simulink model "sm_car_testrig_susp_splitla_shockf_hp"  (R2026a)
settings: Solver=ode23t  StopTime=1e-9  MaxStep=1e-3  AbsTol=1e-4  EnableMultiTasking=on
PostLoadFcn:
  | sm_car_load_vehicle_data(bdroot,'032');
undefined symbols (not defined in the file): Init, UAf, UAr, Vehicle, X, Y, Z
libraries: sm_lib x125, nesl_utility x73, Linkage_Arms x8, Suspension_Utilities x6, fl_lib x4, Linkage_SpLA_S2LAF x2, Linkage_Shock x2, Linkage_Uprights x2
(part 2 of 5)

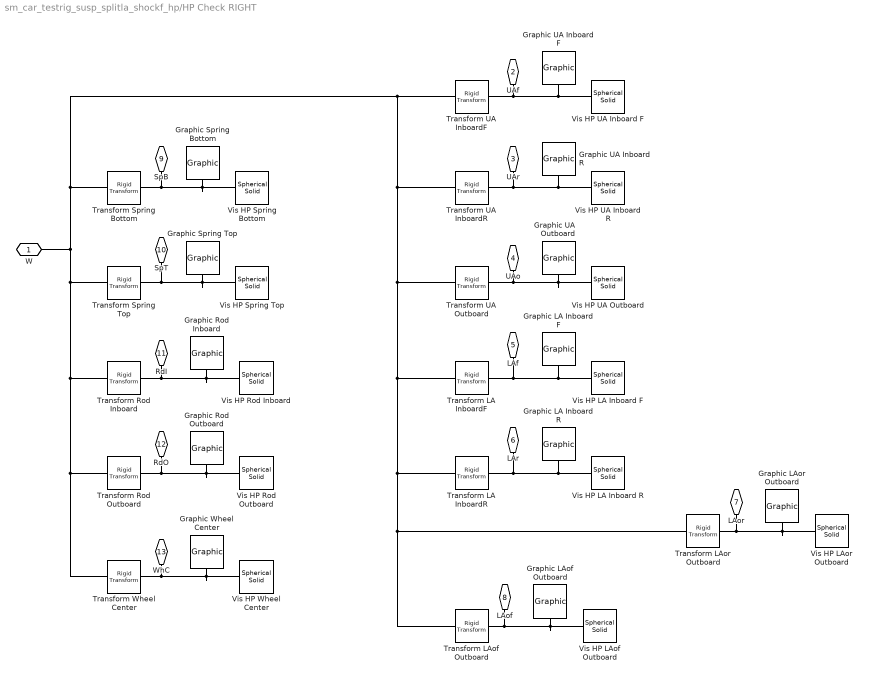
== system sm_car_testrig_susp_splitla_shockf_hp/HP Check RIGHT ==
  Graphic LA Inboard F : sm_lib/Body Elements/Graphic  GraphicType=Marker  MarkerShape=Frame  MarkerSize=size_frm_vis  GraphicVisPropType=SimpleVisualProperties  GraphicDiffuseColor=clr_frm_vis  GraphicOpacity=opc_frm_vis  GraphicSpecularColor=[0.5 0.5 0.5 1.0]  GraphicAmbientColor=[0.15 0.15 0.15 1.0]  GraphicEmissiveColor=[0.0 0.0 0.0 1.0]  GraphicShininess=75
  Graphic LA Inboard R : sm_lib/Body Elements/Graphic  GraphicType=Marker  MarkerShape=Frame  MarkerSize=size_frm_vis  GraphicVisPropType=SimpleVisualProperties  GraphicDiffuseColor=clr_frm_vis  GraphicOpacity=opc_frm_vis  GraphicSpecularColor=[0.5 0.5 0.5 1.0]  GraphicAmbientColor=[0.15 0.15 0.15 1.0]  GraphicEmissiveColor=[0.0 0.0 0.0 1.0]  GraphicShininess=75
  Graphic LAof Outboard : sm_lib/Body Elements/Graphic  GraphicType=Marker  MarkerShape=Frame  MarkerSize=size_frm_vis  GraphicVisPropType=SimpleVisualProperties  GraphicDiffuseColor=clr_frm_vis  GraphicOpacity=opc_frm_vis  GraphicSpecularColor=[0.5 0.5 0.5 1.0]  GraphicAmbientColor=[0.15 0.15 0.15 1.0]  GraphicEmissiveColor=[0.0 0.0 0.0 1.0]  GraphicShininess=75
  Graphic LAor Outboard : sm_lib/Body Elements/Graphic  GraphicType=Marker  MarkerShape=Frame  MarkerSize=size_frm_vis  GraphicVisPropType=SimpleVisualProperties  GraphicDiffuseColor=clr_frm_vis  GraphicOpacity=opc_frm_vis  GraphicSpecularColor=[0.5 0.5 0.5 1.0]  GraphicAmbientColor=[0.15 0.15 0.15 1.0]  GraphicEmissiveColor=[0.0 0.0 0.0 1.0]  GraphicShininess=75
  Graphic Rod Inboard : sm_lib/Body Elements/Graphic  GraphicType=Marker  MarkerShape=Frame  MarkerSize=size_frm_vis  GraphicVisPropType=SimpleVisualProperties  GraphicDiffuseColor=clr_frm_vis  GraphicOpacity=opc_frm_vis  GraphicSpecularColor=[0.5 0.5 0.5 1.0]  GraphicAmbientColor=[0.15 0.15 0.15 1.0]  GraphicEmissiveColor=[0.0 0.0 0.0 1.0]  GraphicShininess=75
  Graphic Rod Outboard : sm_lib/Body Elements/Graphic  GraphicType=Marker  MarkerShape=Frame  MarkerSize=size_frm_vis  GraphicVisPropType=SimpleVisualProperties  GraphicDiffuseColor=clr_frm_vis  GraphicOpacity=opc_frm_vis  GraphicSpecularColor=[0.5 0.5 0.5 1.0]  GraphicAmbientColor=[0.15 0.15 0.15 1.0]  GraphicEmissiveColor=[0.0 0.0 0.0 1.0]  GraphicShininess=75
  Graphic Spring Bottom : sm_lib/Body Elements/Graphic  GraphicType=Marker  MarkerShape=Frame  MarkerSize=size_frm_vis  GraphicVisPropType=SimpleVisualProperties  GraphicDiffuseColor=clr_frm_vis  GraphicOpacity=opc_frm_vis  GraphicSpecularColor=[0.5 0.5 0.5 1.0]  GraphicAmbientColor=[0.15 0.15 0.15 1.0]  GraphicEmissiveColor=[0.0 0.0 0.0 1.0]  GraphicShininess=75
  Graphic Spring Top : sm_lib/Body Elements/Graphic  GraphicType=Marker  MarkerShape=Frame  MarkerSize=size_frm_vis  GraphicVisPropType=SimpleVisualProperties  GraphicDiffuseColor=clr_frm_vis  GraphicOpacity=opc_frm_vis  GraphicSpecularColor=[0.5 0.5 0.5 1.0]  GraphicAmbientColor=[0.15 0.15 0.15 1.0]  GraphicEmissiveColor=[0.0 0.0 0.0 1.0]  GraphicShininess=75
  Graphic UA Inboard F : sm_lib/Body Elements/Graphic  GraphicType=Marker  MarkerShape=Frame  MarkerSize=size_frm_vis  GraphicVisPropType=SimpleVisualProperties  GraphicDiffuseColor=clr_frm_vis  GraphicOpacity=opc_frm_vis  GraphicSpecularColor=[0.5 0.5 0.5 1.0]  GraphicAmbientColor=[0.15 0.15 0.15 1.0]  GraphicEmissiveColor=[0.0 0.0 0.0 1.0]  GraphicShininess=75
  Graphic UA Inboard R : sm_lib/Body Elements/Graphic  GraphicType=Marker  MarkerShape=Frame  MarkerSize=size_frm_vis  GraphicVisPropType=SimpleVisualProperties  GraphicDiffuseColor=clr_frm_vis  GraphicOpacity=opc_frm_vis  GraphicSpecularColor=[0.5 0.5 0.5 1.0]  GraphicAmbientColor=[0.15 0.15 0.15 1.0]  GraphicEmissiveColor=[0.0 0.0 0.0 1.0]  GraphicShininess=75
  Graphic UA Outboard : sm_lib/Body Elements/Graphic  GraphicType=Marker  MarkerShape=Frame  MarkerSize=size_frm_vis  GraphicVisPropType=SimpleVisualProperties  GraphicDiffuseColor=clr_frm_vis  GraphicOpacity=opc_frm_vis  GraphicSpecularColor=[0.5 0.5 0.5 1.0]  GraphicAmbientColor=[0.15 0.15 0.15 1.0]  GraphicEmissiveColor=[0.0 0.0 0.0 1.0]  GraphicShininess=75
  Graphic Wheel Center : sm_lib/Body Elements/Graphic  GraphicType=Marker  MarkerShape=Frame  MarkerSize=size_frm_vis  GraphicVisPropType=SimpleVisualProperties  GraphicDiffuseColor=clr_frm_vis  GraphicOpacity=opc_frm_vis  GraphicSpecularColor=[0.5 0.5 0.5 1.0]  GraphicAmbientColor=[0.15 0.15 0.15 1.0]  GraphicEmissiveColor=[0.0 0.0 0.0 1.0]  GraphicShininess=75
  Transform LA InboardF : sm_lib/Frames and Transforms/Rigid Transform  RotationMethod=None  FollAlignAxisA=+X  BaseAlignAxisA=+Y  FollAlignAxisB=+Y  BaseAlignAxisB=+Z  RotationStandardAxis=+Z  RotationAngle=0.0  RotationAngleUnits=deg  RotationArbitraryAxis=[0 0 1]  RotationSequenceAxes=FollowerAxes  RotationSequence=XYX  RotationSequenceAngles=[0 0 0]  RotationSequenceAnglesUnits=deg  RotationMatrix=[1 0 0; 0 1 0; 0 0 1]  Quaternion=[1 0 0 0]  TranslationMethod=Cartesian  TranslationCartesianOffset=Linkage.LowerArmF.sInboard.Value.*rhs_hp  TranslationCartesianOffsetUnits=m  TranslationStandardAxis=+Z  TranslationStandardOffset=0  TranslationStandardOffsetUnits=m  TranslationROffset=0  TranslationROffsetUnits=m  TranslationThetaOffset=0  TranslationThetaOffsetUnits=deg  TranslationZOffset=0  TranslationZOffsetUnits=m
      settings: AttributesFormatString=%<TranslationCartesianOffset>
  Transform LA InboardR : sm_lib/Frames and Transforms/Rigid Transform  RotationMethod=None  FollAlignAxisA=+X  BaseAlignAxisA=+Y  FollAlignAxisB=+Y  BaseAlignAxisB=+Z  RotationStandardAxis=+Z  RotationAngle=0.0  RotationAngleUnits=deg  RotationArbitraryAxis=[0 0 1]  RotationSequenceAxes=FollowerAxes  RotationSequence=XYX  RotationSequenceAngles=[0 0 0]  RotationSequenceAnglesUnits=deg  RotationMatrix=[1 0 0; 0 1 0; 0 0 1]  Quaternion=[1 0 0 0]  TranslationMethod=Cartesian  TranslationCartesianOffset=Linkage.LowerArmR.sInboard.Value.*rhs_hp  TranslationCartesianOffsetUnits=m  TranslationStandardAxis=+Z  TranslationStandardOffset=0  TranslationStandardOffsetUnits=m  TranslationROffset=0  TranslationROffsetUnits=m  TranslationThetaOffset=0  TranslationThetaOffsetUnits=deg  TranslationZOffset=0  TranslationZOffsetUnits=m
      settings: AttributesFormatString=%<TranslationCartesianOffset>
  Transform LAof Outboard : sm_lib/Frames and Transforms/Rigid Transform  RotationMethod=None  FollAlignAxisA=+X  BaseAlignAxisA=+Y  FollAlignAxisB=+Y  BaseAlignAxisB=+Z  RotationStandardAxis=+Z  RotationAngle=0.0  RotationAngleUnits=deg  RotationArbitraryAxis=[0 0 1]  RotationSequenceAxes=FollowerAxes  RotationSequence=XYX  RotationSequenceAngles=[0 0 0]  RotationSequenceAnglesUnits=deg  RotationMatrix=[1 0 0; 0 1 0; 0 0 1]  Quaternion=[1 0 0 0]  TranslationMethod=Cartesian  TranslationCartesianOffset=Linkage.LowerArmF.sOutboard.Value.*rhs_hp  TranslationCartesianOffsetUnits=m  TranslationStandardAxis=+Z  TranslationStandardOffset=0  TranslationStandardOffsetUnits=m  TranslationROffset=0  TranslationROffsetUnits=m  TranslationThetaOffset=0  TranslationThetaOffsetUnits=deg  TranslationZOffset=0  TranslationZOffsetUnits=m
      settings: AttributesFormatString=%<TranslationCartesianOffset>
  Transform LAor Outboard : sm_lib/Frames and Transforms/Rigid Transform  RotationMethod=None  FollAlignAxisA=+X  BaseAlignAxisA=+Y  FollAlignAxisB=+Y  BaseAlignAxisB=+Z  RotationStandardAxis=+Z  RotationAngle=0.0  RotationAngleUnits=deg  RotationArbitraryAxis=[0 0 1]  RotationSequenceAxes=FollowerAxes  RotationSequence=XYX  RotationSequenceAngles=[0 0 0]  RotationSequenceAnglesUnits=deg  RotationMatrix=[1 0 0; 0 1 0; 0 0 1]  Quaternion=[1 0 0 0]  TranslationMethod=Cartesian  TranslationCartesianOffset=Linkage.LowerArmR.sOutboard.Value.*rhs_hp  TranslationCartesianOffsetUnits=m  TranslationStandardAxis=+Z  TranslationStandardOffset=0  TranslationStandardOffsetUnits=m  TranslationROffset=0  TranslationROffsetUnits=m  TranslationThetaOffset=0  TranslationThetaOffsetUnits=deg  TranslationZOffset=0  TranslationZOffsetUnits=m
      settings: AttributesFormatString=%<TranslationCartesianOffset>
  Transform Rod Inboard : sm_lib/Frames and Transforms/Rigid Transform  RotationMethod=None  FollAlignAxisA=+X  BaseAlignAxisA=+Y  FollAlignAxisB=+Y  BaseAlignAxisB=+Z  RotationStandardAxis=+Z  RotationAngle=0.0  RotationAngleUnits=deg  RotationArbitraryAxis=[0 0 1]  RotationSequenceAxes=FollowerAxes  RotationSequence=XYX  RotationSequenceAngles=[0 0 0]  RotationSequenceAnglesUnits=deg  RotationMatrix=[1 0 0; 0 1 0; 0 0 1]  Quaternion=[1 0 0 0]  TranslationMethod=Cartesian  TranslationCartesianOffset=Linkage.TrackRod.sInboard.Value.*rhs_hp  TranslationCartesianOffsetUnits=m  TranslationStandardAxis=+Z  TranslationStandardOffset=0  TranslationStandardOffsetUnits=m  TranslationROffset=0  TranslationROffsetUnits=m  TranslationThetaOffset=0  TranslationThetaOffsetUnits=deg  TranslationZOffset=0  TranslationZOffsetUnits=m
      settings: AttributesFormatString=%<TranslationCartesianOffset>
  Transform Rod Outboard : sm_lib/Frames and Transforms/Rigid Transform  RotationMethod=None  FollAlignAxisA=+X  BaseAlignAxisA=+Y  FollAlignAxisB=+Y  BaseAlignAxisB=+Z  RotationStandardAxis=+Z  RotationAngle=0.0  RotationAngleUnits=deg  RotationArbitraryAxis=[0 0 1]  RotationSequenceAxes=FollowerAxes  RotationSequence=XYX  RotationSequenceAngles=[0 0 0]  RotationSequenceAnglesUnits=deg  RotationMatrix=[1 0 0; 0 1 0; 0 0 1]  Quaternion=[1 0 0 0]  TranslationMethod=Cartesian  TranslationCartesianOffset=Linkage.TrackRod.sOutboard.Value.*rhs_hp  TranslationCartesianOffsetUnits=m  TranslationStandardAxis=+Z  TranslationStandardOffset=0  TranslationStandardOffsetUnits=m  TranslationROffset=0  TranslationROffsetUnits=m  TranslationThetaOffset=0  TranslationThetaOffsetUnits=deg  TranslationZOffset=0  TranslationZOffsetUnits=m
      settings: AttributesFormatString=%<TranslationCartesianOffset>
  Transform Spring Bottom : sm_lib/Frames and Transforms/Rigid Transform  RotationMethod=None  FollAlignAxisA=+X  BaseAlignAxisA=+Y  FollAlignAxisB=+Y  BaseAlignAxisB=+Z  RotationStandardAxis=+Z  RotationAngle=0.0  RotationAngleUnits=deg  RotationArbitraryAxis=[0 0 1]  RotationSequenceAxes=FollowerAxes  RotationSequence=XYX  RotationSequenceAngles=[0 0 0]  RotationSequenceAnglesUnits=deg  RotationMatrix=[1 0 0; 0 1 0; 0 0 1]  Quaternion=[1 0 0 0]  TranslationMethod=Cartesian  TranslationCartesianOffset=Linkage.Shock.sBottom.Value.*rhs_hp  TranslationCartesianOffsetUnits=m  TranslationStandardAxis=+Z  TranslationStandardOffset=0  TranslationStandardOffsetUnits=m  TranslationROffset=0  TranslationROffsetUnits=m  TranslationThetaOffset=0  TranslationThetaOffsetUnits=deg  TranslationZOffset=0  TranslationZOffsetUnits=m
      settings: AttributesFormatString=%<TranslationCartesianOffset>
  Transform Spring Top : sm_lib/Frames and Transforms/Rigid Transform  RotationMethod=None  FollAlignAxisA=+X  BaseAlignAxisA=+Y  FollAlignAxisB=+Y  BaseAlignAxisB=+Z  RotationStandardAxis=+Z  RotationAngle=0.0  RotationAngleUnits=deg  RotationArbitraryAxis=[0 0 1]  RotationSequenceAxes=FollowerAxes  RotationSequence=XYX  RotationSequenceAngles=[0 0 0]  RotationSequenceAnglesUnits=deg  RotationMatrix=[1 0 0; 0 1 0; 0 0 1]  Quaternion=[1 0 0 0]  TranslationMethod=Cartesian  TranslationCartesianOffset=Linkage.Shock.sTop.Value.*rhs_hp  TranslationCartesianOffsetUnits=m  TranslationStandardAxis=+Z  TranslationStandardOffset=0  TranslationStandardOffsetUnits=m  TranslationROffset=0  TranslationROffsetUnits=m  TranslationThetaOffset=0  TranslationThetaOffsetUnits=deg  TranslationZOffset=0  TranslationZOffsetUnits=m
      settings: AttributesFormatString=%<TranslationCartesianOffset>
  Transform UA InboardF : sm_lib/Frames and Transforms/Rigid Transform  RotationMethod=None  FollAlignAxisA=+X  BaseAlignAxisA=+Y  FollAlignAxisB=+Y  BaseAlignAxisB=+Z  RotationStandardAxis=+Z  RotationAngle=0.0  RotationAngleUnits=deg  RotationArbitraryAxis=[0 0 1]  RotationSequenceAxes=FollowerAxes  RotationSequence=XYX  RotationSequenceAngles=[0 0 0]  RotationSequenceAnglesUnits=deg  RotationMatrix=[1 0 0; 0 1 0; 0 0 1]  Quaternion=[1 0 0 0]  TranslationMethod=Cartesian  TranslationCartesianOffset=Linkage.UpperWishbone.sInboardF.Value.*rhs_hp  TranslationCartesianOffsetUnits=m  TranslationStandardAxis=+Z  TranslationStandardOffset=0  TranslationStandardOffsetUnits=m  TranslationROffset=0  TranslationROffsetUnits=m  TranslationThetaOffset=0  TranslationThetaOffsetUnits=deg  TranslationZOffset=0  TranslationZOffsetUnits=m
      settings: AttributesFormatString=%<TranslationCartesianOffset>
  Transform UA InboardR : sm_lib/Frames and Transforms/Rigid Transform  RotationMethod=None  FollAlignAxisA=+X  BaseAlignAxisA=+Y  FollAlignAxisB=+Y  BaseAlignAxisB=+Z  RotationStandardAxis=+Z  RotationAngle=0.0  RotationAngleUnits=deg  RotationArbitraryAxis=[0 0 1]  RotationSequenceAxes=FollowerAxes  RotationSequence=XYX  RotationSequenceAngles=[0 0 0]  RotationSequenceAnglesUnits=deg  RotationMatrix=[1 0 0; 0 1 0; 0 0 1]  Quaternion=[1 0 0 0]  TranslationMethod=Cartesian  TranslationCartesianOffset=Linkage.UpperWishbone.sInboardR.Value.*rhs_hp  TranslationCartesianOffsetUnits=m  TranslationStandardAxis=+Z  TranslationStandardOffset=0  TranslationStandardOffsetUnits=m  TranslationROffset=0  TranslationROffsetUnits=m  TranslationThetaOffset=0  TranslationThetaOffsetUnits=deg  TranslationZOffset=0  TranslationZOffsetUnits=m
      settings: AttributesFormatString=%<TranslationCartesianOffset>
  Transform UA Outboard : sm_lib/Frames and Transforms/Rigid Transform  RotationMethod=None  FollAlignAxisA=+X  BaseAlignAxisA=+Y  FollAlignAxisB=+Y  BaseAlignAxisB=+Z  RotationStandardAxis=+Z  RotationAngle=0.0  RotationAngleUnits=deg  RotationArbitraryAxis=[0 0 1]  RotationSequenceAxes=FollowerAxes  RotationSequence=XYX  RotationSequenceAngles=[0 0 0]  RotationSequenceAnglesUnits=deg  RotationMatrix=[1 0 0; 0 1 0; 0 0 1]  Quaternion=[1 0 0 0]  TranslationMethod=Cartesian  TranslationCartesianOffset=Linkage.UpperWishbone.sOutboard.Value.*rhs_hp  TranslationCartesianOffsetUnits=m  TranslationStandardAxis=+Z  TranslationStandardOffset=0  TranslationStandardOffsetUnits=m  TranslationROffset=0  TranslationROffsetUnits=m  TranslationThetaOffset=0  TranslationThetaOffsetUnits=deg  TranslationZOffset=0  TranslationZOffsetUnits=m
      settings: AttributesFormatString=%<TranslationCartesianOffset>
  Transform Wheel Center : sm_lib/Frames and Transforms/Rigid Transform  RotationMethod=None  FollAlignAxisA=+X  BaseAlignAxisA=+Y  FollAlignAxisB=+Y  BaseAlignAxisB=+Z  RotationStandardAxis=+Z  RotationAngle=0.0  RotationAngleUnits=deg  RotationArbitraryAxis=[0 0 1]  RotationSequenceAxes=FollowerAxes  RotationSequence=XYX  RotationSequenceAngles=[0 0 0]  RotationSequenceAnglesUnits=deg  RotationMatrix=[1 0 0; 0 1 0; 0 0 1]  Quaternion=[1 0 0 0]  TranslationMethod=Cartesian  TranslationCartesianOffset=Linkage.Upright.sWheelCentre.Value.*rhs_hp  TranslationCartesianOffsetUnits=m  TranslationStandardAxis=+Z  TranslationStandardOffset=0  TranslationStandardOffsetUnits=m  TranslationROffset=0  TranslationROffsetUnits=m  TranslationThetaOffset=0  TranslationThetaOffsetUnits=deg  TranslationZOffset=0  TranslationZOffsetUnits=m
      settings: AttributesFormatString=%<TranslationCartesianOffset>
  Vis HP LA Inboard F : sm_lib/Body Elements/Spherical Solid  SphereRadius=rad_vis_sph  SphereRadiusUnits=m  ExportEntireGeometry=off  InertiaType=CalculateFromGeometry  BasedOnType=Density  Density=1000  DensityUnits=kg/m^3  Mass=1  MassUnits=kg  CenterOfMass=[0 0 0]  CenterOfMassUnits=m  MomentsOfInertia=[1 1 1]  MomentsOfInertiaUnits=kg*m^2  ProductsOfInertia=[0 0 0]  ProductsOfInertiaUnits=kg*m^2  GraphicType=FromGeometry  MarkerShape=Sphere  MarkerSize=10  GraphicVisPropType=SimpleVisualProperties  GraphicDiffuseColor=clr_vis_sph  GraphicOpacity=opc_vis_sph  GraphicSpecularColor=[0.5 0.5 0.5 1.0]  GraphicAmbientColor=[0.15 0.15 0.15 1.0]  GraphicEmissiveColor=[0.0 0.0 0.0 1.0]  GraphicShininess=75  DoExposeReferenceFrame=on  SerializedFrames=<Frames/>
  Vis HP LA Inboard R : sm_lib/Body Elements/Spherical Solid  SphereRadius=rad_vis_sph  SphereRadiusUnits=m  ExportEntireGeometry=off  InertiaType=CalculateFromGeometry  BasedOnType=Density  Density=1000  DensityUnits=kg/m^3  Mass=1  MassUnits=kg  CenterOfMass=[0 0 0]  CenterOfMassUnits=m  MomentsOfInertia=[1 1 1]  MomentsOfInertiaUnits=kg*m^2  ProductsOfInertia=[0 0 0]  ProductsOfInertiaUnits=kg*m^2  GraphicType=FromGeometry  MarkerShape=Sphere  MarkerSize=10  GraphicVisPropType=SimpleVisualProperties  GraphicDiffuseColor=clr_vis_sph  GraphicOpacity=opc_vis_sph  GraphicSpecularColor=[0.5 0.5 0.5 1.0]  GraphicAmbientColor=[0.15 0.15 0.15 1.0]  GraphicEmissiveColor=[0.0 0.0 0.0 1.0]  GraphicShininess=75  DoExposeReferenceFrame=on  SerializedFrames=<Frames/>
  Vis HP LAof Outboard : sm_lib/Body Elements/Spherical Solid  SphereRadius=rad_vis_sph  SphereRadiusUnits=m  ExportEntireGeometry=off  InertiaType=CalculateFromGeometry  BasedOnType=Density  Density=1000  DensityUnits=kg/m^3  Mass=1  MassUnits=kg  CenterOfMass=[0 0 0]  CenterOfMassUnits=m  MomentsOfInertia=[1 1 1]  MomentsOfInertiaUnits=kg*m^2  ProductsOfInertia=[0 0 0]  ProductsOfInertiaUnits=kg*m^2  GraphicType=FromGeometry  MarkerShape=Sphere  MarkerSize=10  GraphicVisPropType=SimpleVisualProperties  GraphicDiffuseColor=clr_vis_sph  GraphicOpacity=opc_vis_sph  GraphicSpecularColor=[0.5 0.5 0.5 1.0]  GraphicAmbientColor=[0.15 0.15 0.15 1.0]  GraphicEmissiveColor=[0.0 0.0 0.0 1.0]  GraphicShininess=75  DoExposeReferenceFrame=on  SerializedFrames=<Frames/>
  Vis HP LAor Outboard : sm_lib/Body Elements/Spherical Solid  SphereRadius=rad_vis_sph  SphereRadiusUnits=m  ExportEntireGeometry=off  InertiaType=CalculateFromGeometry  BasedOnType=Density  Density=1000  DensityUnits=kg/m^3  Mass=1  MassUnits=kg  CenterOfMass=[0 0 0]  CenterOfMassUnits=m  MomentsOfInertia=[1 1 1]  MomentsOfInertiaUnits=kg*m^2  ProductsOfInertia=[0 0 0]  ProductsOfInertiaUnits=kg*m^2  GraphicType=FromGeometry  MarkerShape=Sphere  MarkerSize=10  GraphicVisPropType=SimpleVisualProperties  GraphicDiffuseColor=clr_vis_sph  GraphicOpacity=opc_vis_sph  GraphicSpecularColor=[0.5 0.5 0.5 1.0]  GraphicAmbientColor=[0.15 0.15 0.15 1.0]  GraphicEmissiveColor=[0.0 0.0 0.0 1.0]  GraphicShininess=75  DoExposeReferenceFrame=on  SerializedFrames=<Frames/>
  Vis HP Rod Inboard : sm_lib/Body Elements/Spherical Solid  SphereRadius=rad_vis_sph  SphereRadiusUnits=m  ExportEntireGeometry=off  InertiaType=CalculateFromGeometry  BasedOnType=Density  Density=1000  DensityUnits=kg/m^3  Mass=1  MassUnits=kg  CenterOfMass=[0 0 0]  CenterOfMassUnits=m  MomentsOfInertia=[1 1 1]  MomentsOfInertiaUnits=kg*m^2  ProductsOfInertia=[0 0 0]  ProductsOfInertiaUnits=kg*m^2  GraphicType=FromGeometry  MarkerShape=Sphere  MarkerSize=10  GraphicVisPropType=SimpleVisualProperties  GraphicDiffuseColor=clr_vis_sph  GraphicOpacity=opc_vis_sph  GraphicSpecularColor=[0.5 0.5 0.5 1.0]  GraphicAmbientColor=[0.15 0.15 0.15 1.0]  GraphicEmissiveColor=[0.0 0.0 0.0 1.0]  GraphicShininess=75  DoExposeReferenceFrame=on  SerializedFrames=<Frames/>
  Vis HP Rod Outboard : sm_lib/Body Elements/Spherical Solid  SphereRadius=rad_vis_sph  SphereRadiusUnits=m  ExportEntireGeometry=off  InertiaType=CalculateFromGeometry  BasedOnType=Density  Density=1000  DensityUnits=kg/m^3  Mass=1  MassUnits=kg  CenterOfMass=[0 0 0]  CenterOfMassUnits=m  MomentsOfInertia=[1 1 1]  MomentsOfInertiaUnits=kg*m^2  ProductsOfInertia=[0 0 0]  ProductsOfInertiaUnits=kg*m^2  GraphicType=FromGeometry  MarkerShape=Sphere  MarkerSize=10  GraphicVisPropType=SimpleVisualProperties  GraphicDiffuseColor=clr_vis_sph  GraphicOpacity=opc_vis_sph  GraphicSpecularColor=[0.5 0.5 0.5 1.0]  GraphicAmbientColor=[0.15 0.15 0.15 1.0]  GraphicEmissiveColor=[0.0 0.0 0.0 1.0]  GraphicShininess=75  DoExposeReferenceFrame=on  SerializedFrames=<Frames/>
  Vis HP Spring Bottom : sm_lib/Body Elements/Spherical Solid  SphereRadius=rad_vis_sph  SphereRadiusUnits=m  ExportEntireGeometry=off  InertiaType=CalculateFromGeometry  BasedOnType=Density  Density=1000  DensityUnits=kg/m^3  Mass=1  MassUnits=kg  CenterOfMass=[0 0 0]  CenterOfMassUnits=m  MomentsOfInertia=[1 1 1]  MomentsOfInertiaUnits=kg*m^2  ProductsOfInertia=[0 0 0]  ProductsOfInertiaUnits=kg*m^2  GraphicType=FromGeometry  MarkerShape=Sphere  MarkerSize=10  GraphicVisPropType=SimpleVisualProperties  GraphicDiffuseColor=clr_vis_sph  GraphicOpacity=opc_vis_sph  GraphicSpecularColor=[0.5 0.5 0.5 1.0]  GraphicAmbientColor=[0.15 0.15 0.15 1.0]  GraphicEmissiveColor=[0.0 0.0 0.0 1.0]  GraphicShininess=75  DoExposeReferenceFrame=on  SerializedFrames=<Frames/>
  Vis HP Spring Top : sm_lib/Body Elements/Spherical Solid  SphereRadius=rad_vis_sph  SphereRadiusUnits=m  ExportEntireGeometry=off  InertiaType=CalculateFromGeometry  BasedOnType=Density  Density=1000  DensityUnits=kg/m^3  Mass=1  MassUnits=kg  CenterOfMass=[0 0 0]  CenterOfMassUnits=m  MomentsOfInertia=[1 1 1]  MomentsOfInertiaUnits=kg*m^2  ProductsOfInertia=[0 0 0]  ProductsOfInertiaUnits=kg*m^2  GraphicType=FromGeometry  MarkerShape=Sphere  MarkerSize=10  GraphicVisPropType=SimpleVisualProperties  GraphicDiffuseColor=clr_vis_sph  GraphicOpacity=opc_vis_sph  GraphicSpecularColor=[0.5 0.5 0.5 1.0]  GraphicAmbientColor=[0.15 0.15 0.15 1.0]  GraphicEmissiveColor=[0.0 0.0 0.0 1.0]  GraphicShininess=75  DoExposeReferenceFrame=on  SerializedFrames=<Frames/>
  Vis HP UA Inboard F : sm_lib/Body Elements/Spherical Solid  SphereRadius=rad_vis_sph  SphereRadiusUnits=m  ExportEntireGeometry=off  InertiaType=CalculateFromGeometry  BasedOnType=Density  Density=1000  DensityUnits=kg/m^3  Mass=1  MassUnits=kg  CenterOfMass=[0 0 0]  CenterOfMassUnits=m  MomentsOfInertia=[1 1 1]  MomentsOfInertiaUnits=kg*m^2  ProductsOfInertia=[0 0 0]  ProductsOfInertiaUnits=kg*m^2  GraphicType=FromGeometry  MarkerShape=Sphere  MarkerSize=10  GraphicVisPropType=SimpleVisualProperties  GraphicDiffuseColor=clr_vis_sph  GraphicOpacity=opc_vis_sph  GraphicSpecularColor=[0.5 0.5 0.5 1.0]  GraphicAmbientColor=[0.15 0.15 0.15 1.0]  GraphicEmissiveColor=[0.0 0.0 0.0 1.0]  GraphicShininess=75  DoExposeReferenceFrame=on  SerializedFrames=<Frames/>
  Vis HP UA Inboard R : sm_lib/Body Elements/Spherical Solid  SphereRadius=rad_vis_sph  SphereRadiusUnits=m  ExportEntireGeometry=off  InertiaType=CalculateFromGeometry  BasedOnType=Density  Density=1000  DensityUnits=kg/m^3  Mass=1  MassUnits=kg  CenterOfMass=[0 0 0]  CenterOfMassUnits=m  MomentsOfInertia=[1 1 1]  MomentsOfInertiaUnits=kg*m^2  ProductsOfInertia=[0 0 0]  ProductsOfInertiaUnits=kg*m^2  GraphicType=FromGeometry  MarkerShape=Sphere  MarkerSize=10  GraphicVisPropType=SimpleVisualProperties  GraphicDiffuseColor=clr_vis_sph  GraphicOpacity=opc_vis_sph  GraphicSpecularColor=[0.5 0.5 0.5 1.0]  GraphicAmbientColor=[0.15 0.15 0.15 1.0]  GraphicEmissiveColor=[0.0 0.0 0.0 1.0]  GraphicShininess=75  DoExposeReferenceFrame=on  SerializedFrames=<Frames/>
  Vis HP UA Outboard : sm_lib/Body Elements/Spherical Solid  SphereRadius=rad_vis_sph  SphereRadiusUnits=m  ExportEntireGeometry=off  InertiaType=CalculateFromGeometry  BasedOnType=Density  Density=1000  DensityUnits=kg/m^3  Mass=1  MassUnits=kg  CenterOfMass=[0 0 0]  CenterOfMassUnits=m  MomentsOfInertia=[1 1 1]  MomentsOfInertiaUnits=kg*m^2  ProductsOfInertia=[0 0 0]  ProductsOfInertiaUnits=kg*m^2  GraphicType=FromGeometry  MarkerShape=Sphere  MarkerSize=10  GraphicVisPropType=SimpleVisualProperties  GraphicDiffuseColor=clr_vis_sph  GraphicOpacity=opc_vis_sph  GraphicSpecularColor=[0.5 0.5 0.5 1.0]  GraphicAmbientColor=[0.15 0.15 0.15 1.0]  GraphicEmissiveColor=[0.0 0.0 0.0 1.0]  GraphicShininess=75  DoExposeReferenceFrame=on  SerializedFrames=<Frames/>
  Vis HP Wheel Center : sm_lib/Body Elements/Spherical Solid  SphereRadius=rad_vis_sph  SphereRadiusUnits=m  ExportEntireGeometry=off  InertiaType=CalculateFromGeometry  BasedOnType=Density  Density=1000  DensityUnits=kg/m^3  Mass=1  MassUnits=kg  CenterOfMass=[0 0 0]  CenterOfMassUnits=m  MomentsOfInertia=[1 1 1]  MomentsOfInertiaUnits=kg*m^2  ProductsOfInertia=[0 0 0]  ProductsOfInertiaUnits=kg*m^2  GraphicType=FromGeometry  MarkerShape=Sphere  MarkerSize=10  GraphicVisPropType=SimpleVisualProperties  GraphicDiffuseColor=clr_vis_sph  GraphicOpacity=opc_vis_sph  GraphicSpecularColor=[0.5 0.5 0.5 1.0]  GraphicAmbientColor=[0.15 0.15 0.15 1.0]  GraphicEmissiveColor=[0.0 0.0 0.0 1.0]  GraphicShininess=75  DoExposeReferenceFrame=on  SerializedFrames=<Frames/>
  W : PMIOPort  Side=Left
  UAf : PMIOPort  Port=2  Side=Right
  UAr : PMIOPort  Port=3  Side=Right
  UAo : PMIOPort  Port=4  Side=Right
  LAf : PMIOPort  Port=5  Side=Right
  LAr : PMIOPort  Port=6  Side=Right
  LAor : PMIOPort  Port=7  Side=Right
  LAof : PMIOPort  Port=8  Side=Right
  SpB : PMIOPort  Port=9  Side=Right
  SpT : PMIOPort  Port=10  Side=Right
  RdI : PMIOPort  Port=11  Side=Right
  RdO : PMIOPort  Port=12  Side=Right
  WhC : PMIOPort  Port=13  Side=Right
  connections:
  LAor/RConn1 -- Transform LAor Outboard/RConn1 -- Graphic LAor Outboard/RConn1 -- Vis HP LAor Outboard/RConn1
  Transform Rod Inboard/RConn1 -- RdI/RConn1 -- Vis HP Rod Inboard/RConn1 -- Graphic Rod Inboard/RConn1
  Vis HP LA Inboard R/RConn1 -- Transform LA InboardR/RConn1 -- LAr/RConn1 -- Graphic LA Inboard R/RConn1
  Vis HP LA Inboard F/RConn1 -- Graphic LA Inboard F/RConn1 -- LAf/RConn1 -- Transform LA InboardF/RConn1
  Vis HP UA Inboard R/RConn1 -- Transform UA InboardR/RConn1 -- UAr/RConn1 -- Graphic UA Inboard R/RConn1
  Vis HP UA Inboard F/RConn1 -- Graphic UA Inboard F/RConn1 -- UAf/RConn1 -- Transform UA InboardF/RConn1
  Vis HP Wheel Center/RConn1 -- Transform Wheel Center/RConn1 -- WhC/RConn1 -- Graphic Wheel Center/RConn1
  Vis HP Rod Outboard/RConn1 -- Transform Rod Outboard/RConn1 -- RdO/RConn1 -- Graphic Rod Outboard/RConn1
  Graphic LAof Outboard/RConn1 -- Transform LAof Outboard/RConn1 -- LAof/RConn1 -- Vis HP LAof Outboard/RConn1
  Graphic Spring Bottom/RConn1 -- Transform Spring Bottom/RConn1 -- SpB/RConn1 -- Vis HP Spring Bottom/RConn1
  Graphic UA Outboard/RConn1 -- Vis HP UA Outboard/RConn1 -- UAo/RConn1 -- Transform UA Outboard/RConn1
  Transform LA InboardF/LConn1 -- Transform LA InboardR/LConn1 -- Transform LAof Outboard/LConn1 -- Transform LAor Outboard/LConn1 -- Transform UA InboardF/LConn1 -- Transform Spring Bottom/LConn1 -- Transform Spring Top/LConn1 -- Transform Rod Inboard/LConn1 -- Transform Rod Outboard/LConn1 -- Transform Wheel Center/LConn1 -- W/RConn1 -- Transform UA InboardR/LConn1 -- Transform UA Outboard/LConn1
  Vis HP Spring Top/RConn1 -- Transform Spring Top/RConn1 -- SpT/RConn1 -- Graphic Spring Top/RConn1

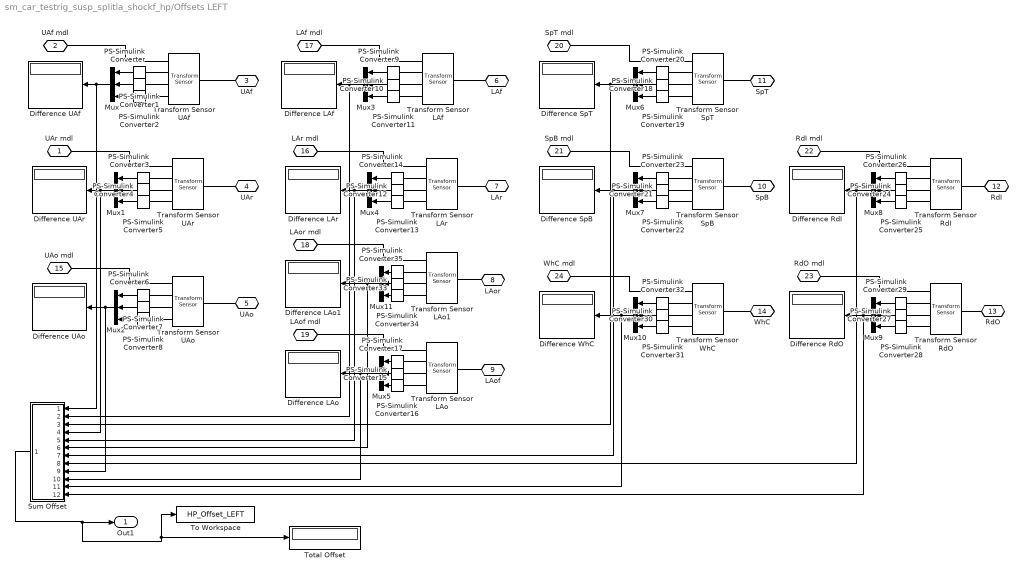
== system sm_car_testrig_susp_splitla_shockf_hp/Offsets LEFT ==
  Difference LAf : Display
  Difference LAo : Display
  Difference LAo1 : Display
  Difference LAr : Display
  Difference RdI : Display
  Difference RdO : Display
  Difference SpB : Display
  Difference SpT : Display
  Difference UAf : Display
  Difference UAo : Display
  Difference UAr : Display
  Difference WhC : Display
  Mux{,1..11} (12 alike) : Mux  Inputs=3
  PS-Simulink Converter{,1..35} (36 alike) : nesl_utility/PS-Simulink Converter  PhysicalDomain=network_engine_domain  SubClassName=ps_output  LeftPortType=input  RightPortType=output  PseudoPeriodic=off  Frequencies=[]  VectorFormat=1-D array  Unit=1  AffineConversion=off
  Sum Offset : Subsystem
  To Workspace : ToWorkspace  VariableName=HP_Offset_LEFT  SaveFormat=Timeseries  SampleTime=-1
  Total Offset : Display
  Transform Sensor LAf : sm_lib/Frames and Transforms/Transform Sensor  MeasurementFrame=World  RotationSequence=XYX  SenseAngle=off  SenseAxis=off  SenseQ=off  SenseR=off  SenseRotationSequence=off  SenseOmegaX=off  SenseOmegaY=off  SenseOmegaZ=off  SenseOmega=off  SenseQDot=off  SenseRDot=off  SenseRotationSequenceDot=off  SenseAlphaX=off  SenseAlphaY=off  SenseAlphaZ=off  SenseAlpha=off  SenseQDDot=off  SenseRDDot=off  SenseX=on  SenseY=on  SenseZ=on  SenseXYZ=off  SenseRad=off  SenseAzim=off  SenseDist=off  SenseInc=off  SenseXDot=off  SenseYDot=off  SenseZDot=off  SenseXYZDot=off  SenseRadDot=off  SenseAzimDot=off  SenseDistDot=off  SenseIncDot=off  SenseXDDot=off  SenseYDDot=off  SenseZDDot=off  SenseXYZDDot=off  SenseRadDDot=off  SenseAzimDDot=off  SenseDistDDot=off  SenseIncDDot=off
  Transform Sensor LAo : sm_lib/Frames and Transforms/Transform Sensor  MeasurementFrame=World  RotationSequence=XYX  SenseAngle=off  SenseAxis=off  SenseQ=off  SenseR=off  SenseRotationSequence=off  SenseOmegaX=off  SenseOmegaY=off  SenseOmegaZ=off  SenseOmega=off  SenseQDot=off  SenseRDot=off  SenseRotationSequenceDot=off  SenseAlphaX=off  SenseAlphaY=off  SenseAlphaZ=off  SenseAlpha=off  SenseQDDot=off  SenseRDDot=off  SenseX=on  SenseY=on  SenseZ=on  SenseXYZ=off  SenseRad=off  SenseAzim=off  SenseDist=off  SenseInc=off  SenseXDot=off  SenseYDot=off  SenseZDot=off  SenseXYZDot=off  SenseRadDot=off  SenseAzimDot=off  SenseDistDot=off  SenseIncDot=off  SenseXDDot=off  SenseYDDot=off  SenseZDDot=off  SenseXYZDDot=off  SenseRadDDot=off  SenseAzimDDot=off  SenseDistDDot=off  SenseIncDDot=off
  Transform Sensor LAo1 : sm_lib/Frames and Transforms/Transform Sensor  MeasurementFrame=World  RotationSequence=XYX  SenseAngle=off  SenseAxis=off  SenseQ=off  SenseR=off  SenseRotationSequence=off  SenseOmegaX=off  SenseOmegaY=off  SenseOmegaZ=off  SenseOmega=off  SenseQDot=off  SenseRDot=off  SenseRotationSequenceDot=off  SenseAlphaX=off  SenseAlphaY=off  SenseAlphaZ=off  SenseAlpha=off  SenseQDDot=off  SenseRDDot=off  SenseX=on  SenseY=on  SenseZ=on  SenseXYZ=off  SenseRad=off  SenseAzim=off  SenseDist=off  SenseInc=off  SenseXDot=off  SenseYDot=off  SenseZDot=off  SenseXYZDot=off  SenseRadDot=off  SenseAzimDot=off  SenseDistDot=off  SenseIncDot=off  SenseXDDot=off  SenseYDDot=off  SenseZDDot=off  SenseXYZDDot=off  SenseRadDDot=off  SenseAzimDDot=off  SenseDistDDot=off  SenseIncDDot=off
  Transform Sensor LAr : sm_lib/Frames and Transforms/Transform Sensor  MeasurementFrame=World  RotationSequence=XYX  SenseAngle=off  SenseAxis=off  SenseQ=off  SenseR=off  SenseRotationSequence=off  SenseOmegaX=off  SenseOmegaY=off  SenseOmegaZ=off  SenseOmega=off  SenseQDot=off  SenseRDot=off  SenseRotationSequenceDot=off  SenseAlphaX=off  SenseAlphaY=off  SenseAlphaZ=off  SenseAlpha=off  SenseQDDot=off  SenseRDDot=off  SenseX=on  SenseY=on  SenseZ=on  SenseXYZ=off  SenseRad=off  SenseAzim=off  SenseDist=off  SenseInc=off  SenseXDot=off  SenseYDot=off  SenseZDot=off  SenseXYZDot=off  SenseRadDot=off  SenseAzimDot=off  SenseDistDot=off  SenseIncDot=off  SenseXDDot=off  SenseYDDot=off  SenseZDDot=off  SenseXYZDDot=off  SenseRadDDot=off  SenseAzimDDot=off  SenseDistDDot=off  SenseIncDDot=off
  Transform Sensor RdI : sm_lib/Frames and Transforms/Transform Sensor  MeasurementFrame=World  RotationSequence=XYX  SenseAngle=off  SenseAxis=off  SenseQ=off  SenseR=off  SenseRotationSequence=off  SenseOmegaX=off  SenseOmegaY=off  SenseOmegaZ=off  SenseOmega=off  SenseQDot=off  SenseRDot=off  SenseRotationSequenceDot=off  SenseAlphaX=off  SenseAlphaY=off  SenseAlphaZ=off  SenseAlpha=off  SenseQDDot=off  SenseRDDot=off  SenseX=on  SenseY=on  SenseZ=on  SenseXYZ=off  SenseRad=off  SenseAzim=off  SenseDist=off  SenseInc=off  SenseXDot=off  SenseYDot=off  SenseZDot=off  SenseXYZDot=off  SenseRadDot=off  SenseAzimDot=off  SenseDistDot=off  SenseIncDot=off  SenseXDDot=off  SenseYDDot=off  SenseZDDot=off  SenseXYZDDot=off  SenseRadDDot=off  SenseAzimDDot=off  SenseDistDDot=off  SenseIncDDot=off
  Transform Sensor RdO : sm_lib/Frames and Transforms/Transform Sensor  MeasurementFrame=World  RotationSequence=XYX  SenseAngle=off  SenseAxis=off  SenseQ=off  SenseR=off  SenseRotationSequence=off  SenseOmegaX=off  SenseOmegaY=off  SenseOmegaZ=off  SenseOmega=off  SenseQDot=off  SenseRDot=off  SenseRotationSequenceDot=off  SenseAlphaX=off  SenseAlphaY=off  SenseAlphaZ=off  SenseAlpha=off  SenseQDDot=off  SenseRDDot=off  SenseX=on  SenseY=on  SenseZ=on  SenseXYZ=off  SenseRad=off  SenseAzim=off  SenseDist=off  SenseInc=off  SenseXDot=off  SenseYDot=off  SenseZDot=off  SenseXYZDot=off  SenseRadDot=off  SenseAzimDot=off  SenseDistDot=off  SenseIncDot=off  SenseXDDot=off  SenseYDDot=off  SenseZDDot=off  SenseXYZDDot=off  SenseRadDDot=off  SenseAzimDDot=off  SenseDistDDot=off  SenseIncDDot=off
  Transform Sensor SpB : sm_lib/Frames and Transforms/Transform Sensor  MeasurementFrame=World  RotationSequence=XYX  SenseAngle=off  SenseAxis=off  SenseQ=off  SenseR=off  SenseRotationSequence=off  SenseOmegaX=off  SenseOmegaY=off  SenseOmegaZ=off  SenseOmega=off  SenseQDot=off  SenseRDot=off  SenseRotationSequenceDot=off  SenseAlphaX=off  SenseAlphaY=off  SenseAlphaZ=off  SenseAlpha=off  SenseQDDot=off  SenseRDDot=off  SenseX=on  SenseY=on  SenseZ=on  SenseXYZ=off  SenseRad=off  SenseAzim=off  SenseDist=off  SenseInc=off  SenseXDot=off  SenseYDot=off  SenseZDot=off  SenseXYZDot=off  SenseRadDot=off  SenseAzimDot=off  SenseDistDot=off  SenseIncDot=off  SenseXDDot=off  SenseYDDot=off  SenseZDDot=off  SenseXYZDDot=off  SenseRadDDot=off  SenseAzimDDot=off  SenseDistDDot=off  SenseIncDDot=off
  Transform Sensor SpT : sm_lib/Frames and Transforms/Transform Sensor  MeasurementFrame=World  RotationSequence=XYX  SenseAngle=off  SenseAxis=off  SenseQ=off  SenseR=off  SenseRotationSequence=off  SenseOmegaX=off  SenseOmegaY=off  SenseOmegaZ=off  SenseOmega=off  SenseQDot=off  SenseRDot=off  SenseRotationSequenceDot=off  SenseAlphaX=off  SenseAlphaY=off  SenseAlphaZ=off  SenseAlpha=off  SenseQDDot=off  SenseRDDot=off  SenseX=on  SenseY=on  SenseZ=on  SenseXYZ=off  SenseRad=off  SenseAzim=off  SenseDist=off  SenseInc=off  SenseXDot=off  SenseYDot=off  SenseZDot=off  SenseXYZDot=off  SenseRadDot=off  SenseAzimDot=off  SenseDistDot=off  SenseIncDot=off  SenseXDDot=off  SenseYDDot=off  SenseZDDot=off  SenseXYZDDot=off  SenseRadDDot=off  SenseAzimDDot=off  SenseDistDDot=off  SenseIncDDot=off
  Transform Sensor UAf : sm_lib/Frames and Transforms/Transform Sensor  MeasurementFrame=World  RotationSequence=XYX  SenseAngle=off  SenseAxis=off  SenseQ=off  SenseR=off  SenseRotationSequence=off  SenseOmegaX=off  SenseOmegaY=off  SenseOmegaZ=off  SenseOmega=off  SenseQDot=off  SenseRDot=off  SenseRotationSequenceDot=off  SenseAlphaX=off  SenseAlphaY=off  SenseAlphaZ=off  SenseAlpha=off  SenseQDDot=off  SenseRDDot=off  SenseX=on  SenseY=on  SenseZ=on  SenseXYZ=off  SenseRad=off  SenseAzim=off  SenseDist=off  SenseInc=off  SenseXDot=off  SenseYDot=off  SenseZDot=off  SenseXYZDot=off  SenseRadDot=off  SenseAzimDot=off  SenseDistDot=off  SenseIncDot=off  SenseXDDot=off  SenseYDDot=off  SenseZDDot=off  SenseXYZDDot=off  SenseRadDDot=off  SenseAzimDDot=off  SenseDistDDot=off  SenseIncDDot=off
  Transform Sensor UAo : sm_lib/Frames and Transforms/Transform Sensor  MeasurementFrame=World  RotationSequence=XYX  SenseAngle=off  SenseAxis=off  SenseQ=off  SenseR=off  SenseRotationSequence=off  SenseOmegaX=off  SenseOmegaY=off  SenseOmegaZ=off  SenseOmega=off  SenseQDot=off  SenseRDot=off  SenseRotationSequenceDot=off  SenseAlphaX=off  SenseAlphaY=off  SenseAlphaZ=off  SenseAlpha=off  SenseQDDot=off  SenseRDDot=off  SenseX=on  SenseY=on  SenseZ=on  SenseXYZ=off  SenseRad=off  SenseAzim=off  SenseDist=off  SenseInc=off  SenseXDot=off  SenseYDot=off  SenseZDot=off  SenseXYZDot=off  SenseRadDot=off  SenseAzimDot=off  SenseDistDot=off  SenseIncDot=off  SenseXDDot=off  SenseYDDot=off  SenseZDDot=off  SenseXYZDDot=off  SenseRadDDot=off  SenseAzimDDot=off  SenseDistDDot=off  SenseIncDDot=off
  Transform Sensor UAr : sm_lib/Frames and Transforms/Transform Sensor  MeasurementFrame=World  RotationSequence=XYX  SenseAngle=off  SenseAxis=off  SenseQ=off  SenseR=off  SenseRotationSequence=off  SenseOmegaX=off  SenseOmegaY=off  SenseOmegaZ=off  SenseOmega=off  SenseQDot=off  SenseRDot=off  SenseRotationSequenceDot=off  SenseAlphaX=off  SenseAlphaY=off  SenseAlphaZ=off  SenseAlpha=off  SenseQDDot=off  SenseRDDot=off  SenseX=on  SenseY=on  SenseZ=on  SenseXYZ=off  SenseRad=off  SenseAzim=off  SenseDist=off  SenseInc=off  SenseXDot=off  SenseYDot=off  SenseZDot=off  SenseXYZDot=off  SenseRadDot=off  SenseAzimDot=off  SenseDistDot=off  SenseIncDot=off  SenseXDDot=off  SenseYDDot=off  SenseZDDot=off  SenseXYZDDot=off  SenseRadDDot=off  SenseAzimDDot=off  SenseDistDDot=off  SenseIncDDot=off
  Transform Sensor WhC : sm_lib/Frames and Transforms/Transform Sensor  MeasurementFrame=World  RotationSequence=XYX  SenseAngle=off  SenseAxis=off  SenseQ=off  SenseR=off  SenseRotationSequence=off  SenseOmegaX=off  SenseOmegaY=off  SenseOmegaZ=off  SenseOmega=off  SenseQDot=off  SenseRDot=off  SenseRotationSequenceDot=off  SenseAlphaX=off  SenseAlphaY=off  SenseAlphaZ=off  SenseAlpha=off  SenseQDDot=off  SenseRDDot=off  SenseX=on  SenseY=on  SenseZ=on  SenseXYZ=off  SenseRad=off  SenseAzim=off  SenseDist=off  SenseInc=off  SenseXDot=off  SenseYDot=off  SenseZDot=off  SenseXYZDot=off  SenseRadDot=off  SenseAzimDot=off  SenseDistDot=off  SenseIncDot=off  SenseXDDot=off  SenseYDDot=off  SenseZDDot=off  SenseXYZDDot=off  SenseRadDDot=off  SenseAzimDDot=off  SenseDistDDot=off  SenseIncDDot=off
  UAr mdl : PMIOPort  Side=Right
  UAf mdl : PMIOPort  Port=2  Side=Right
  UAf : PMIOPort  Port=3  Side=Left
  UAr : PMIOPort  Port=4  Side=Left
  UAo : PMIOPort  Port=5  Side=Left
  LAf : PMIOPort  Port=6  Side=Left
  LAr : PMIOPort  Port=7  Side=Left
  LAor : PMIOPort  Port=8  Side=Left
  LAof : PMIOPort  Port=9  Side=Left
  SpB : PMIOPort  Port=10  Side=Left
  SpT : PMIOPort  Port=11  Side=Left
  RdI : PMIOPort  Port=12  Side=Left
  RdO : PMIOPort  Port=13  Side=Left
  WhC : PMIOPort  Port=14  Side=Left
  UAo mdl : PMIOPort  Port=15  Side=Right
  LAr mdl : PMIOPort  Port=16  Side=Right
  LAf mdl : PMIOPort  Port=17  Side=Right
  LAor mdl : PMIOPort  Port=18  Side=Right
  LAof mdl : PMIOPort  Port=19  Side=Right
  SpT mdl : PMIOPort  Port=20  Side=Right
  SpB mdl : PMIOPort  Port=21  Side=Right
  RdI mdl : PMIOPort  Port=22  Side=Right
  RdO mdl : PMIOPort  Port=23  Side=Right
  WhC mdl : PMIOPort  Port=24  Side=Right
  Out1 : Outport  VectorParamsAs1DForOutWhenUnconnected=off
  wires:
  Mux/1 -> Sum Offset/1(In1), Difference UAf/1
  PS-Simulink Converter1/1 -> Mux/2
  PS-Simulink Converter2/1 -> Mux/3
  PS-Simulink Converter/1 -> Mux/1
  PS-Simulink Converter3/1 -> Mux1/1
  PS-Simulink Converter5/1 -> Mux1/3
  PS-Simulink Converter4/1 -> Mux1/2
  Mux1/1 -> Sum Offset/4(In4), Difference UAr/1
  Mux2/1 -> Sum Offset/9(In8), Difference UAo/1
  PS-Simulink Converter7/1 -> Mux2/2
  PS-Simulink Converter8/1 -> Mux2/3
  PS-Simulink Converter6/1 -> Mux2/1
  PS-Simulink Converter9/1 -> Mux3/1
  PS-Simulink Converter11/1 -> Mux3/3
  PS-Simulink Converter10/1 -> Mux3/2
  Mux3/1 -> Sum Offset/2(In2), Difference LAf/1
  Mux4/1 -> Difference LAr/1, Sum Offset/5(In5)
  PS-Simulink Converter12/1 -> Mux4/2
  PS-Simulink Converter13/1 -> Mux4/3
  PS-Simulink Converter14/1 -> Mux4/1
  PS-Simulink Converter17/1 -> Mux5/1
  PS-Simulink Converter16/1 -> Mux5/3
  PS-Simulink Converter15/1 -> Mux5/2
  Mux5/1 -> Sum Offset/10(In9), Difference LAo/1
  Mux6/1 -> Sum Offset/3(In3), Difference SpT/1
  PS-Simulink Converter18/1 -> Mux6/2
  PS-Simulink Converter19/1 -> Mux6/3
  PS-Simulink Converter20/1 -> Mux6/1
  PS-Simulink Converter23/1 -> Mux7/1
  PS-Simulink Converter22/1 -> Mux7/3
  PS-Simulink Converter21/1 -> Mux7/2
  Mux7/1 -> Sum Offset/7(In6), Difference SpB/1
  Mux8/1 -> Sum Offset/8(In7), Difference RdI/1
  PS-Simulink Converter24/1 -> Mux8/2
  PS-Simulink Converter25/1 -> Mux8/3
  PS-Simulink Converter26/1 -> Mux8/1
  PS-Simulink Converter29/1 -> Mux9/1
  PS-Simulink Converter28/1 -> Mux9/3
  PS-Simulink Converter27/1 -> Mux9/2
  Mux9/1 -> Sum Offset/12(In11), Difference RdO/1
  Mux10/1 -> Sum Offset/11(In10), Difference WhC/1
  PS-Simulink Converter30/1 -> Mux10/2
  PS-Simulink Converter31/1 -> Mux10/3
  PS-Simulink Converter32/1 -> Mux10/1
  Sum Offset/1(Out1) -> Total Offset/1, To Workspace/1, Out1/1
  Mux11/1 -> Sum Offset/6(In12), Difference LAo1/1
  PS-Simulink Converter33/1 -> Mux11/2
  PS-Simulink Converter34/1 -> Mux11/3
  PS-Simulink Converter35/1 -> Mux11/1
  connections:
  PS-Simulink Converter2/LConn1 -- Transform Sensor UAf/RConn4
  PS-Simulink Converter1/LConn1 -- Transform Sensor UAf/RConn3
  Transform Sensor UAf/LConn1 -- UAf/RConn1
  Transform Sensor UAf/RConn2 -- PS-Simulink Converter/LConn1
  Transform Sensor UAf/RConn1 -- UAf mdl/RConn1
  UAr mdl/RConn1 -- Transform Sensor UAr/RConn1
  Transform Sensor UAr/RConn2 -- PS-Simulink Converter3/LConn1
  UAr/RConn1 -- Transform Sensor UAr/LConn1
  PS-Simulink Converter4/LConn1 -- Transform Sensor UAr/RConn3
  PS-Simulink Converter5/LConn1 -- Transform Sensor UAr/RConn4
  PS-Simulink Converter7/LConn1 -- Transform Sensor UAo/RConn3
  UAo/RConn1 -- Transform Sensor UAo/LConn1
  PS-Simulink Converter8/LConn1 -- Transform Sensor UAo/RConn4
  UAo mdl/RConn1 -- Transform Sensor UAo/RConn1
  Transform Sensor UAo/RConn2 -- PS-Simulink Converter6/LConn1
  Transform Sensor LAf/RConn1 -- LAf mdl/RConn1
  Transform Sensor LAf/RConn2 -- PS-Simulink Converter9/LConn1
  LAf/RConn1 -- Transform Sensor LAf/LConn1
  PS-Simulink Converter10/LConn1 -- Transform Sensor LAf/RConn3
  PS-Simulink Converter11/LConn1 -- Transform Sensor LAf/RConn4
  PS-Simulink Converter13/LConn1 -- Transform Sensor LAr/RConn4
  PS-Simulink Converter12/LConn1 -- Transform Sensor LAr/RConn3
  Transform Sensor LAr/RConn2 -- PS-Simulink Converter14/LConn1
  Transform Sensor LAr/RConn1 -- LAr mdl/RConn1
  LAr/RConn1 -- Transform Sensor LAr/LConn1
  LAof/RConn1 -- Transform Sensor LAo/LConn1
  PS-Simulink Converter15/LConn1 -- Transform Sensor LAo/RConn3
  PS-Simulink Converter16/LConn1 -- Transform Sensor LAo/RConn4
  Transform Sensor LAo/RConn2 -- PS-Simulink Converter17/LConn1
  Transform Sensor LAo/RConn1 -- LAof mdl/RConn1
  PS-Simulink Converter19/LConn1 -- Transform Sensor SpT/RConn4
  PS-Simulink Converter18/LConn1 -- Transform Sensor SpT/RConn3
  Transform Sensor SpT/RConn2 -- PS-Simulink Converter20/LConn1
  Transform Sensor SpT/RConn1 -- SpT mdl/RConn1
  SpT/RConn1 -- Transform Sensor SpT/LConn1
  SpB/RConn1 -- Transform Sensor SpB/LConn1
  Transform Sensor SpB/RConn2 -- PS-Simulink Converter23/LConn1
  Transform Sensor SpB/RConn1 -- SpB mdl/RConn1
  PS-Simulink Converter21/LConn1 -- Transform Sensor SpB/RConn3
  PS-Simulink Converter22/LConn1 -- Transform Sensor SpB/RConn4
  PS-Simulink Converter25/LConn1 -- Transform Sensor RdI/RConn4
  PS-Simulink Converter24/LConn1 -- Transform Sensor RdI/RConn3
  Transform Sensor RdI/RConn2 -- PS-Simulink Converter26/LConn1
  Transform Sensor RdI/RConn1 -- RdI mdl/RConn1
  RdI/RConn1 -- Transform Sensor RdI/LConn1
  RdO/RConn1 -- Transform Sensor RdO/LConn1
  Transform Sensor RdO/RConn2 -- PS-Simulink Converter29/LConn1
  PS-Simulink Converter27/LConn1 -- Transform Sensor RdO/RConn3
  PS-Simulink Converter28/LConn1 -- Transform Sensor RdO/RConn4
  Transform Sensor RdO/RConn1 -- RdO mdl/RConn1
  PS-Simulink Converter31/LConn1 -- Transform Sensor WhC/RConn4
  PS-Simulink Converter30/LConn1 -- Transform Sensor WhC/RConn3
  Transform Sensor WhC/RConn2 -- PS-Simulink Converter32/LConn1
  Transform Sensor WhC/RConn1 -- WhC mdl/RConn1
  WhC/RConn1 -- Transform Sensor WhC/LConn1
  Transform Sensor LAo1/RConn1 -- LAor mdl/RConn1
  PS-Simulink Converter33/LConn1 -- Transform Sensor LAo1/RConn3
  LAor/RConn1 -- Transform Sensor LAo1/LConn1
  PS-Simulink Converter34/LConn1 -- Transform Sensor LAo1/RConn4
  Transform Sensor LAo1/RConn2 -- PS-Simulink Converter35/LConn1
